simulink model "BCH_sim"  (R2023b)
settings: Solver=VariableStepDiscrete  StartTime=0.0  StopTime=inf  RelTol=1e-3  EnableMultiTasking=on
PreLoadFcn:
  | N = 7;    % Codeword length
  | EbNo = 8; % Default EbNo
  | K = 4;    % Message length
libraries: commblkcod2 x2, commdigbbndpm3 x2, dspstat3 x2, commrandsrc3 x1, commchan3 x1, commsink2 x1
settings Model: Creator=The MathWorks, Inc.  LastModifiedBy=lucas
settings SolverCC: AlgebraicLoopSolver=TrustRegion
settings DataIOCC: LimitDataPoints=on  SaveFormat=Array  ReturnWorkspaceOutputs=off  SignalLoggingName=sigsOut
settings OptimizationCC: ReuseModelBlockBuffer=off  ExpressionDepthLimit=2147483647  InitFltsAndDblsToZero=on  LifeSpan=inf
settings DebuggingCC: SaveWithParameterizedLinksMsg=none  SignalResolutionControl=TryResolveAllWithWarning  MultiTaskDSMMsg=warning  MultiTaskCondExecSysMsg=none  UnconnectedInputMsg=warning  UnconnectedOutputMsg=warning  UnconnectedLineMsg=warning  StateNameClashWarn=warning  SFUnexpectedBacktrackingDiag=warning  SFNoUnconditionalDefaultTransitionDiag=warning  SFExecutionAtInitializationDiag=none  ArithmeticOperatorsInVariantConditions=warning
settings HardwareCC: ProdBitPerPointer=32  ProdBitPerSizeT=32  ProdBitPerPtrDiffT=32  ProdLargestAtomicFloat=None  ProdIntDivRoundTo=Undefined  ProdEndianess=Unspecified  ProdWordSize=32  ProdHWDeviceType=32-bit Generic  TargetUnknown=on
settings ModelReferenceCC: EnableRefExpFcnMdlSchedulingChecks=on  PropagateSignalLabelsOutOfModel=off
settings SFSimCC: SimUseLocalCustomCode=off  CustomCodeUndefinedFunction=UseInterfaceOnly
settings RTWCC: RTWUseLocalCustomCode=off
settings CodeAppCC: StateflowObjectComments=on
settings GRTTargetCC: TargetFcnLib=ansi_tfl_tmw.mat  TargetLangStandard=C89/C90 (ANSI)  CombineOutputUpdateFcns=off  GRTInterface=on
settings ConfigComp: CovMetricSettings=dw  CovSaveCumulativeToWorkspaceVar=on  CovSaveSingleToWorkspaceVar=on  CovExternalEMLEnable=off

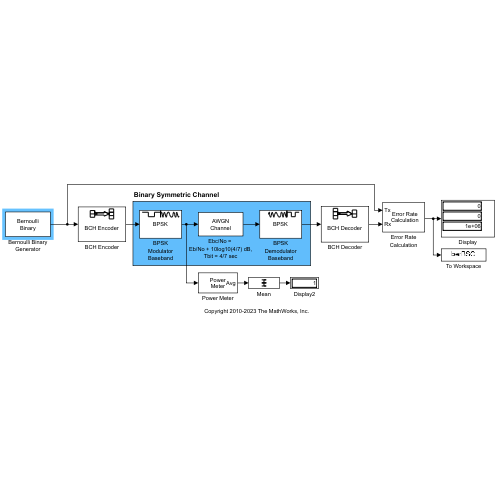
[thumbnail: Simulink's stored preview of the top-level diagram]
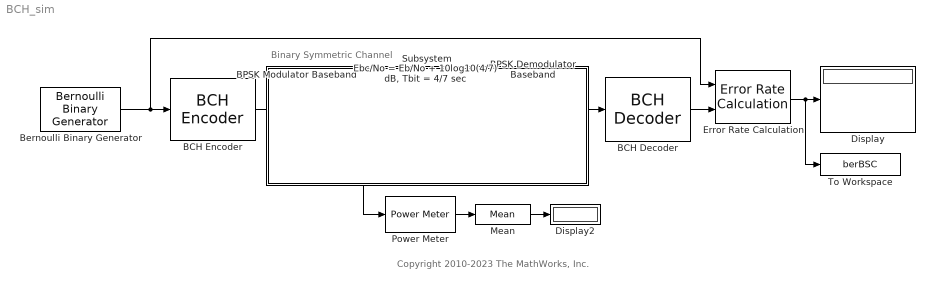
== system BCH_sim ==
  note: Binary Symmetric Channel
  note: Copyright 2010-2023 The MathWorks, Inc.
  BCH Decoder : commblkcod2/BCH Decoder  n=7  k=4  specShortening=off  shortenedK=5  specGenPoly=off  genPoly='X^10 + X^8 + X^5 + X^4 + X^2 + X + 1'  specPrimPoly=off  prPoly='X^4 + X + 1'  specDisableGenCheck=off  specPuncture=off  punctVec=[ones(8,1); zeros(2,1)]  specErasurePort=off  showNumErr=off
  BCH Encoder : commblkcod2/BCH Encoder  n=7  k=4  specShortening=off  shortenedK=5  specGenPoly=off  genPoly='X^10 + X^8 + X^5 + X^4 + X^2 + X + 1'  specPrimPoly=off  prPoly='X^4 + X + 1'  specDisableGenCheck=off  specPuncture=off  punctVec=[ones(8,1); zeros(2,1)]
  BPSK Demodulator Baseband : commdigbbndpm3/BPSK Demodulator Baseband  DecType=Hard decision  VarSource=Dialog  Variance=1  Ph=0  outDtype=Inherit via internal rule  derotateFactorWordLen=16  derotateFactorDataTypeStr=Inherit: Same word length as input  derotateFactorLastDataTypeStr=Inherit: Same word length as input
  BPSK Modulator Baseband : commdigbbndpm3/BPSK Modulator Baseband  Ph=0  outDtype=double  outWordLen=16  outUDDataType=sfix(16)  outFracLenMode=Best precision  outFracLen=15  outDataTypeStr=double  outLastDataTypeStr=double
  Bernoulli Binary Generator : commrandsrc3/Bernoulli Binary Generator  ProbabilityOfZero=0.5  SeedSource=Auto  Seed=0  SampleTime=1  SamplesPerFrame=4  OutputDataType=double  SimulateUsing=Interpreted execution
  Display : Display
  Display2 : Display
  "Ebc/No = Eb/No + 10log10(4/7) dB, Tbit = 4/7 sec" : commchan3/AWGN Channel  LegacyMode=off  NoiseMethod="Signal to noise ratio  (Eb/No)"  noiseMode="Signal to noise ratio  (Eb/No)"  EbNo=EbNo + 10*log10(K/N)  EsNo=6.75 + 10*log10(4/7)  SNR=10  BitsPerSymbol=1  SignalPower=1  SamplesPerSymbol=1  SymbolPeriod=4/7  VarianceSource=Parameter  Variance=1  RandomStream=mt19937ar with seed  Seed=67  SimulateUsing=Code generation
  Error Rate Calculation : commsink2/Error Rate Calculation  N=0  st_delay=0  cp_mode=Entire frame  subframe=[]  PMode=Port  WsName=ErrorVec  RsMode2=off  stop=on  numErr=200  maxBits=1e6
  Mean : dspstat3/Mean  run=off  InputProcessing=Columns as channels (frame based)  reset_popup=None  directionMode=Each column  dimension=1  roiEnable=off  roiType=Rectangles  roiPortion=Entire ROI  roiOutput=Individual statistics for each ROI  roiFlag=off  roundingMode=Floor  overflowMode=off  outputDataTypeStr=Inherit: Same as accumulator  outputMin=[]  outputMax=[]  outputLastDataTypeStr=Inherit: Same as accumulator
  Power Meter : dspstat3/Power Meter  Measurement=Average power  ReferenceLoad=1  OutputPowerUnits=Watts  WindowLength=256  OverlapLength=255  AllowArbitraryInputLength=off  ComputeCCDF=off  PowerRange=50  PowerResolution=0.1  CCDFOutput=Relative power (dB above average power)  ProbabilityVector=[ 10; 1; 0.1; 0.01; 0.001; 0.0001 ]  RelativePowerVector=[ 0; 3; 6; 9; 12 ]  ResetPort=off  SimulateUsing=Code generation
      settings: LibrarySourceBlock=commutil2/Power Meter
  Subsystem : Subsystem
      mask Display: disp('')
  To Workspace : ToWorkspace  VariableName=berBSC  SampleTime=-1
      settings: Save2DSignal=2-D array (concatenate along first dimension)
  wires:
  BPSK Modulator Baseband/1 -> Power Meter/1, "Ebc/No = Eb/No + 10log10(4/7) dB, Tbit = 4/7 sec"/1
  "Ebc/No = Eb/No + 10log10(4/7) dB, Tbit = 4/7 sec"/1 -> BPSK Demodulator Baseband/1
  Error Rate Calculation/1 -> To Workspace/1, Display/1
  Bernoulli Binary Generator/1 -> BCH Encoder/1, Error Rate Calculation/1
  BCH Encoder/1 -> BPSK Modulator Baseband/1
  BPSK Demodulator Baseband/1 -> BCH Decoder/1
  BCH Decoder/1 -> Error Rate Calculation/2
  Power Meter/1 -> Mean/1
  Mean/1 -> Display2/1

== system BCH_sim/Subsystem ==
